simulink model "EOR_Ctrl"  (R2020a)
settings: Solver=FixedStepAuto  StartTime=0.0  StopTime=10.0  FixedStep=DT  RelTol=1e-3  EnableMultiTasking=on
values from neighbouring files (symbols this model uses):
  DT = 0.00625    [run_Top_Model.m]
  N_w = 3    [run_Top_Model.m]
  T_cal = 60    [run_Top_Model.m]
  T_s = 0.1    [run_Top_Model.m]
  tp = turbine_params_5MW()    [baseline_design.m]    (also in run_Top_Model.m)
settings Model: Creator=lpwoolcock  LastModifiedBy=lpwoolcock

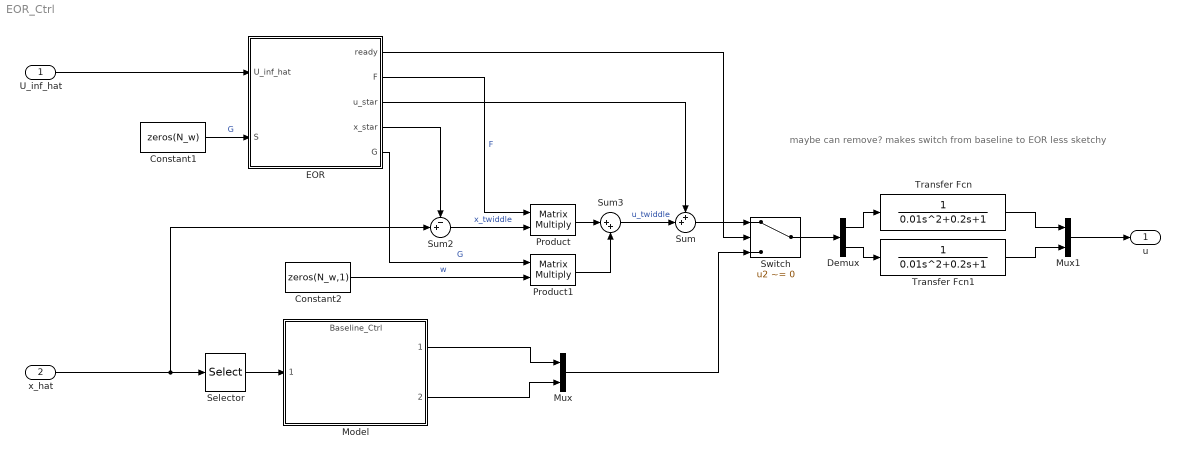
== system EOR_Ctrl ==
  note: maybe can remove? makes switch from baseline to EOR less sketchy
  U_inf_hat : Inport
  x_hat : Inport  Port=2  PortDimensions=5
  Constant1 : Constant  Value=zeros(N_w)
  Constant2 : Constant  Value=zeros(N_w,1)
  Demux : Demux  Outputs=2
  EOR : Stateflow chart  TreatAsAtomicUnit=on
  Model : ModelReference  ModelNameDialog=Baseline_Ctrl.slx  SimulationMode=Normal  ModelReferenceVersion=1.8
  Mux : Mux  Inputs=2
  Mux1 : Mux  Inputs=2
  Product : Product  Multiplication=Matrix(*)
  Product1 : Product  Multiplication=Matrix(*)
  Selector : Selector  InputPortWidth=5  IndexOptions=Index vector (dialog)  Indices=1  OutputSizes=1
  Sum : Sum  Inputs=++|
  Sum2 : Sum  Inputs=-+|
  Sum3 : Sum  Inputs=|++
  Switch : Switch  Criteria=u2 ~= 0
  Transfer Fcn : TransferFcn  Denominator=[0.01 0.2 1]
  Transfer Fcn1 : TransferFcn  Denominator=[0.01 0.2 1]
  u : Outport
  wires:
  Model/1 -> Mux/1
  Model/2 -> Mux/2
  Selector/1 -> Model/1
  Mux/1 -> Switch/3
  Sum/1 -> Switch/1
  EOR/2(F) -> Product/1  "F"
  EOR/1(ready) -> Switch/2
  EOR/3(u_star) -> Sum/1
  Sum2/1 -> Product/2  "x_twiddle"
  EOR/4(x_star) -> Sum2/1
  Mux1/1 -> u/1
  Transfer Fcn1/1 -> Mux1/2
  Transfer Fcn/1 -> Mux1/1
  Switch/1 -> Demux/1
  Demux/1 -> Transfer Fcn/1
  Demux/2 -> Transfer Fcn1/1
  Product1/1 -> Sum3/2
  Product/1 -> Sum3/1
  Sum3/1 -> Sum/2  "u_twiddle"
  Constant1/1 -> EOR/2(S)  "G"
  EOR/5(G) -> Product1/1  "G"
  U_inf_hat/1 -> EOR/1(U_inf_hat)
  x_hat/1 -> Selector/1, Sum2/2
  Constant2/1 -> Product1/2  "w"

== stateflow chart EOR_Ctrl/EOR ==
  state Calibrate
    during:
    if ~isnan(U_inf_hat)
    n = n+1;
    v_x0 = v_x0 + U_inf_hat*DT/T_cal;
    end
  state Region_2
    entry:
    [x_star, u_star, ~, ~, ~, ~, K2] = eq_region2(tp,v_x0, T_s);
    F = [0 0 0 0 0; -K2 0 0];
    ready = 1;
  state Region_3
    entry:
    [x_star, u_star, A3, B3, C3, H3, K3] = eq_region3(tp,v_x0, T_s);
    F = [-K3;0 0 0 0 0];
    E_w3(1) = H3(1);
    D_ew3(1) = fdiff(@(vx) interp1(tp.v_x_bp, tp.theta_v_x, vx, 'pchip'),...
    v_x0);
    [Pi3, Gamma3] = eor_solve(A3, B3, E_w3, C3, 0, D_ew3, S);
    G(1,:) = Gamma3 + K3*Pi3;
    ready = 1;
    during:
    [Pi3, Gamma3] = eor_solve(A3, B3, E_w3, C3, 0, D_ew3, S);
    G(1,:) = Gamma3 + K3*Pi3;
  (default) -> Calibrate
  Calibrate -> Region_2 [order 2] : [n*DT>T_cal & v_x0<=tp.v_x_rated]
  Calibrate -> Region_3 [order 1] : [n*DT>T_cal & v_x0>tp.v_x_rated]
  data: U_inf_hat input; ready output =0; F output size=[2 5] =zeros(2,5); u_star output size=[2 1] =zeros(2,1); x_star output size=5 =zeros(5,1); n local =0; DT parameter; v_x0 local =0; tp parameter; T_s parameter; T_cal parameter; K2 local =zeros(1,3); K3 local =zeros(1,5); A3 local size=[5 5] =zeros(5,5); B3 local size=[5 1] =zeros(5,1); C3 local size=[1 5] =zeros(1,5); H3 local size=[5 1] =zeros(5,1); N_w parameter size=1; S input size=[N_w N_w]; G output size=[2 N_w] =zeros(2,N_w); D_ew3 local size=[1 N_w] =zeros(1,N_w); E_w3 local size=[5 N_w] =zeros(5,N_w); Pi3 local size=[5 N_w] =zeros(5, N_w); Gamma3 local size=[1 N_w] =zeros(1, N_w)
